simulink model "grid_traditional"  (R2023b)
settings: Solver=ode23s  StartTime=0.0  StopTime=32  RelTol=1e-3
values from neighbouring files (symbols this model uses):
  Ts = 5e-6    (= 5e-06)    [model_parameters.m]
undefined symbols (not defined in the file or in its folder): gcbh, Grid, IBR, L, SG, sps_rtmsupport, TX
libraries: spsThreePhaseVIMeasurementLib x13, spsFourierLib x13, spsPowerPositiveSequenceLib x13, spsThreePhaseSeriesRLCLoadLib x11, spsThreePhaseSeriesRLCBranchLib x10, spsThreePhaseTransformerTwoWindingsLib x10, spsDCVoltageSourceLib x8, spsFirstOrderFilterLib x8, spsabctodq0Lib x8, spsSimplifiedSynchronousMachinepuUnitsLib x6, spsGroundLib x4, spsUniversalBridgeLib x4
(part 2 of 2)

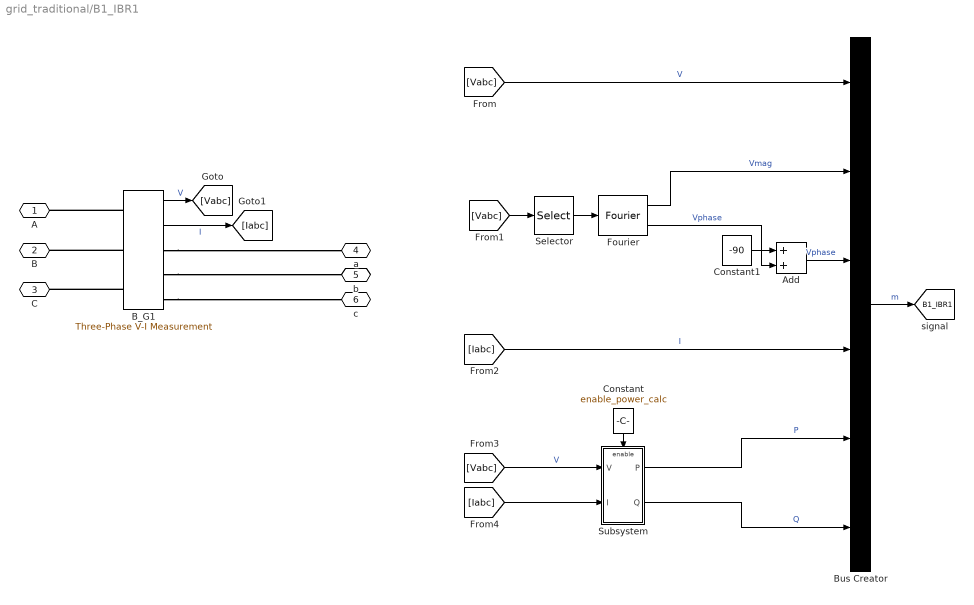
== system grid_traditional/B1_IBR1 ==
  Add : Sum
  B_G1 : spsThreePhaseVIMeasurementLib/Three-Phase V-I Measurement  VoltageMeasurement=phase-to-ground  SetLabelV=off  LabelV=G1_Vabc  Vpu=on  VpuLL=off  CurrentMeasurement=yes  SetLabelI=off  LabelI=G1_Iabc  Ipu=on  Pbase=Sbase  Vbase=Vbase  OutputType=Complex  PhasorSimulation=off  PSBequivalent=0
  Bus Creator : BusCreator  Inputs=6
  Constant : Constant  Value=enable_power_calc  OutDataTypeStr=boolean
  Constant1 : Constant  Value=-90
  Fourier : spsFourierLib/Fourier  Freq=f  n=1  InInit=[0, 0]  Ts=Ts
  Selector : Selector  InputPortWidth=3  IndexOptions=Index vector (dialog)  Indices=[1]  OutputSizes=1
  Subsystem : Subsystem
  A : PMIOPort  Side=Left
  B : PMIOPort  Port=2  Side=Left
  C : PMIOPort  Port=3  Side=Left
  a : PMIOPort  Port=4  Side=Right
  b : PMIOPort  Port=5  Side=Right
  c : PMIOPort  Port=6  Side=Right
  tag scope: B1_IBR1=global
  wires:
  Selector/1 -> Fourier/1
  Bus Creator/1 -> [B1_IBR1]  "m"
  Constant/1 -> Subsystem/Enable
  Subsystem/1(P) -> Bus Creator/5  "P"
  Subsystem/2(Q) -> Bus Creator/6  "Q"
  Fourier/1 -> Bus Creator/2  "Vmag"
  B_G1/1 -> [Vabc]  "V"
  [Vabc] -> Bus Creator/1  "V"
  [Vabc] -> Selector/1
  B_G1/2 -> [Iabc]  "I"
  [Iabc] -> Bus Creator/4  "I"
  [Vabc] -> Subsystem/1(V)  "V"
  [Iabc] -> Subsystem/2(I)
  Add/1 -> Bus Creator/3  "Vphase"
  Fourier/2 -> Add/2  "Vphase"
  Constant1/1 -> Add/1
  connections:
  B_G1/LConn1 -- A/RConn1
  B_G1/LConn3 -- C/RConn1
  B_G1/RConn2 -- b/RConn1
  B_G1/RConn1 -- a/RConn1
  B_G1/LConn2 -- B/RConn1
  B_G1/RConn3 -- c/RConn1

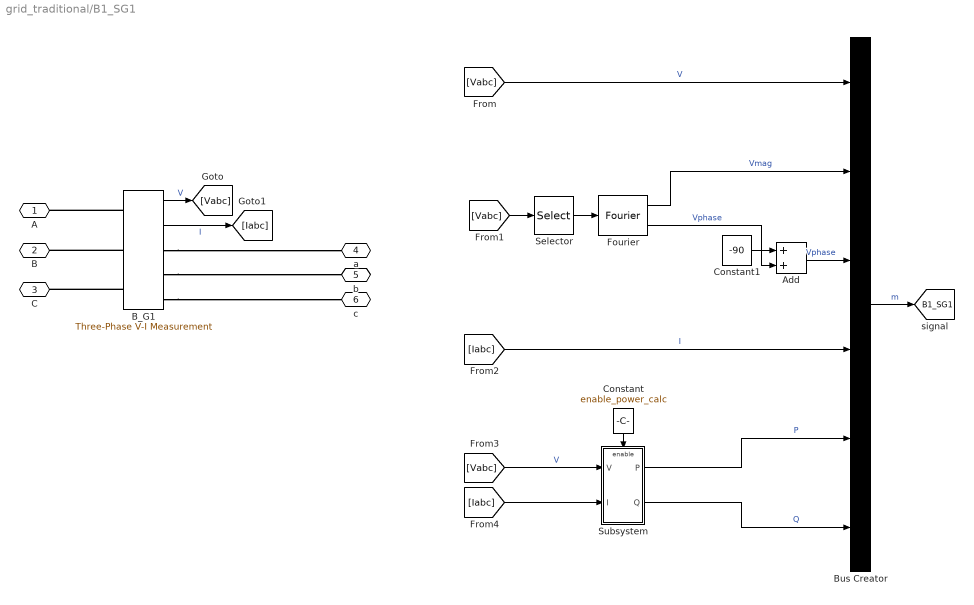
== system grid_traditional/B1_SG1 ==
  Add : Sum
  B_G1 : spsThreePhaseVIMeasurementLib/Three-Phase V-I Measurement  VoltageMeasurement=phase-to-ground  SetLabelV=off  LabelV=G1_Vabc  Vpu=on  VpuLL=off  CurrentMeasurement=yes  SetLabelI=off  LabelI=G1_Iabc  Ipu=on  Pbase=Sbase  Vbase=Vbase  OutputType=Complex  PhasorSimulation=off  PSBequivalent=0
  Bus Creator : BusCreator  Inputs=6
  Constant : Constant  Value=enable_power_calc  OutDataTypeStr=boolean
  Constant1 : Constant  Value=-90
  Fourier : spsFourierLib/Fourier  Freq=f  n=1  InInit=[0, 0]  Ts=Ts
  Selector : Selector  InputPortWidth=3  IndexOptions=Index vector (dialog)  Indices=[1]  OutputSizes=1
  Subsystem : Subsystem
  A : PMIOPort  Side=Left
  B : PMIOPort  Port=2  Side=Left
  C : PMIOPort  Port=3  Side=Left
  a : PMIOPort  Port=4  Side=Right
  b : PMIOPort  Port=5  Side=Right
  c : PMIOPort  Port=6  Side=Right
  tag scope: B1_SG1=global
  wires:
  Selector/1 -> Fourier/1
  Bus Creator/1 -> [B1_SG1]  "m"
  Constant/1 -> Subsystem/Enable
  Subsystem/1(P) -> Bus Creator/5  "P"
  Subsystem/2(Q) -> Bus Creator/6  "Q"
  Fourier/1 -> Bus Creator/2  "Vmag"
  B_G1/1 -> [Vabc]  "V"
  [Vabc] -> Bus Creator/1  "V"
  [Vabc] -> Selector/1
  B_G1/2 -> [Iabc]  "I"
  [Iabc] -> Bus Creator/4  "I"
  [Vabc] -> Subsystem/1(V)  "V"
  [Iabc] -> Subsystem/2(I)
  Add/1 -> Bus Creator/3  "Vphase"
  Fourier/2 -> Add/2  "Vphase"
  Constant1/1 -> Add/1
  connections:
  B_G1/LConn1 -- A/RConn1
  B_G1/LConn3 -- C/RConn1
  B_G1/RConn2 -- b/RConn1
  B_G1/RConn1 -- a/RConn1
  B_G1/LConn2 -- B/RConn1
  B_G1/RConn3 -- c/RConn1

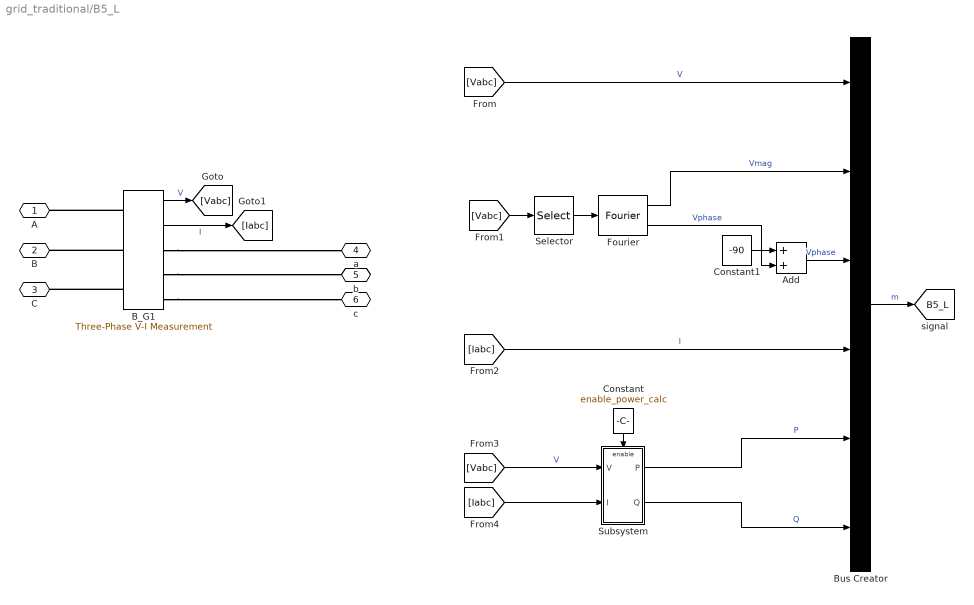
== system grid_traditional/B5_L ==
  Add : Sum
  B_G1 : spsThreePhaseVIMeasurementLib/Three-Phase V-I Measurement  VoltageMeasurement=phase-to-ground  SetLabelV=off  LabelV=G1_Vabc  Vpu=on  VpuLL=off  CurrentMeasurement=yes  SetLabelI=off  LabelI=G1_Iabc  Ipu=on  Pbase=Sbase  Vbase=Vbase  OutputType=Complex  PhasorSimulation=off  PSBequivalent=0
  Bus Creator : BusCreator  Inputs=6
  Constant : Constant  Value=enable_power_calc  OutDataTypeStr=boolean
  Constant1 : Constant  Value=-90
  Fourier : spsFourierLib/Fourier  Freq=f  n=1  InInit=[0, 0]  Ts=Ts
  Selector : Selector  InputPortWidth=3  IndexOptions=Index vector (dialog)  Indices=[1]  OutputSizes=1
  Subsystem : Subsystem
  A : PMIOPort  Side=Left
  B : PMIOPort  Port=2  Side=Left
  C : PMIOPort  Port=3  Side=Left
  a : PMIOPort  Port=4  Side=Right
  b : PMIOPort  Port=5  Side=Right
  c : PMIOPort  Port=6  Side=Right
  tag scope: B5_L=global
  wires:
  Selector/1 -> Fourier/1
  Bus Creator/1 -> [B5_L]  "m"
  Constant/1 -> Subsystem/Enable
  Subsystem/1(P) -> Bus Creator/5  "P"
  Subsystem/2(Q) -> Bus Creator/6  "Q"
  Fourier/1 -> Bus Creator/2  "Vmag"
  B_G1/1 -> [Vabc]  "V"
  [Vabc] -> Bus Creator/1  "V"
  [Vabc] -> Selector/1
  B_G1/2 -> [Iabc]  "I"
  [Iabc] -> Bus Creator/4  "I"
  [Vabc] -> Subsystem/1(V)  "V"
  [Iabc] -> Subsystem/2(I)
  Add/1 -> Bus Creator/3  "Vphase"
  Fourier/2 -> Add/2  "Vphase"
  Constant1/1 -> Add/1
  connections:
  B_G1/LConn1 -- A/RConn1
  B_G1/LConn3 -- C/RConn1
  B_G1/RConn2 -- b/RConn1
  B_G1/RConn1 -- a/RConn1
  B_G1/LConn2 -- B/RConn1
  B_G1/RConn3 -- c/RConn1

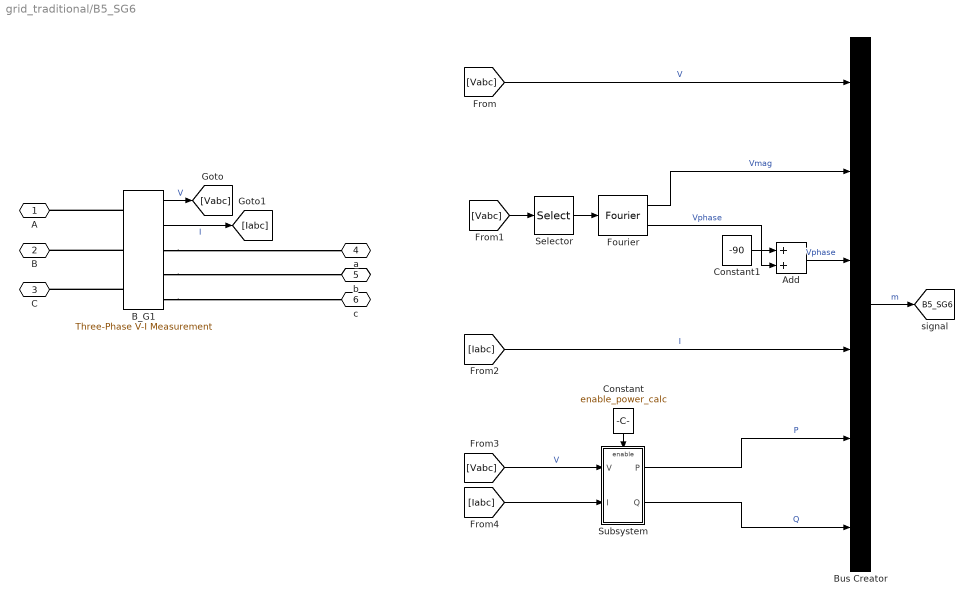
== system grid_traditional/B5_SG6 ==
  Add : Sum
  B_G1 : spsThreePhaseVIMeasurementLib/Three-Phase V-I Measurement  VoltageMeasurement=phase-to-ground  SetLabelV=off  LabelV=G1_Vabc  Vpu=on  VpuLL=off  CurrentMeasurement=yes  SetLabelI=off  LabelI=G1_Iabc  Ipu=on  Pbase=Sbase  Vbase=Vbase  OutputType=Complex  PhasorSimulation=off  PSBequivalent=0
  Bus Creator : BusCreator  Inputs=6
  Constant : Constant  Value=enable_power_calc  OutDataTypeStr=boolean
  Constant1 : Constant  Value=-90
  Fourier : spsFourierLib/Fourier  Freq=f  n=1  InInit=[0, 0]  Ts=Ts
  Selector : Selector  InputPortWidth=3  IndexOptions=Index vector (dialog)  Indices=[1]  OutputSizes=1
  Subsystem : Subsystem
  A : PMIOPort  Side=Left
  B : PMIOPort  Port=2  Side=Left
  C : PMIOPort  Port=3  Side=Left
  a : PMIOPort  Port=4  Side=Right
  b : PMIOPort  Port=5  Side=Right
  c : PMIOPort  Port=6  Side=Right
  tag scope: B5_SG6=global
  wires:
  Selector/1 -> Fourier/1
  Bus Creator/1 -> [B5_SG6]  "m"
  Constant/1 -> Subsystem/Enable
  Subsystem/1(P) -> Bus Creator/5  "P"
  Subsystem/2(Q) -> Bus Creator/6  "Q"
  Fourier/1 -> Bus Creator/2  "Vmag"
  B_G1/1 -> [Vabc]  "V"
  [Vabc] -> Bus Creator/1  "V"
  [Vabc] -> Selector/1
  B_G1/2 -> [Iabc]  "I"
  [Iabc] -> Bus Creator/4  "I"
  [Vabc] -> Subsystem/1(V)  "V"
  [Iabc] -> Subsystem/2(I)
  Add/1 -> Bus Creator/3  "Vphase"
  Fourier/2 -> Add/2  "Vphase"
  Constant1/1 -> Add/1
  connections:
  B_G1/LConn1 -- A/RConn1
  B_G1/LConn3 -- C/RConn1
  B_G1/RConn2 -- b/RConn1
  B_G1/RConn1 -- a/RConn1
  B_G1/LConn2 -- B/RConn1
  B_G1/RConn3 -- c/RConn1

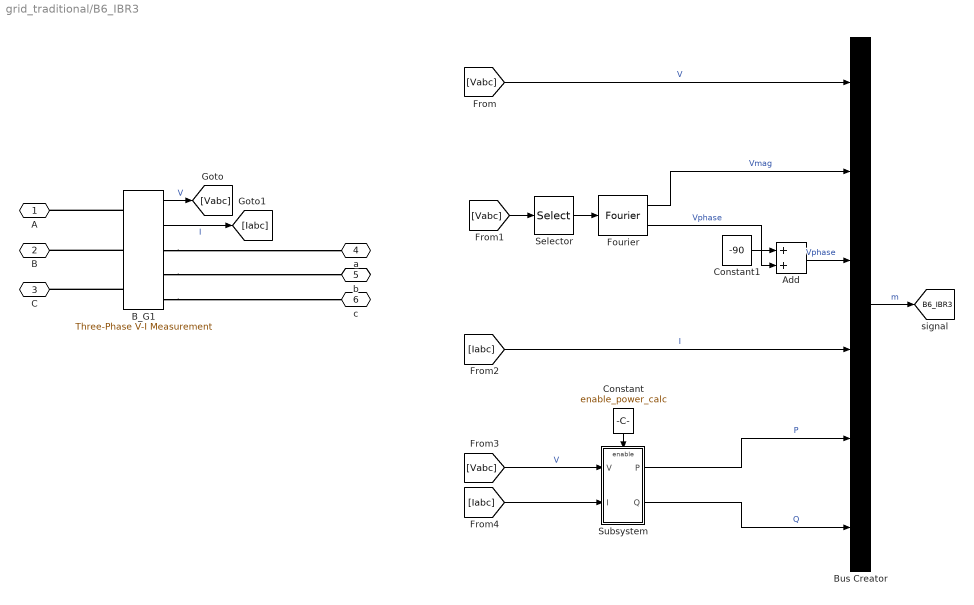
== system grid_traditional/B6_IBR3 ==
  Add : Sum
  B_G1 : spsThreePhaseVIMeasurementLib/Three-Phase V-I Measurement  VoltageMeasurement=phase-to-ground  SetLabelV=off  LabelV=G1_Vabc  Vpu=on  VpuLL=off  CurrentMeasurement=yes  SetLabelI=off  LabelI=G1_Iabc  Ipu=on  Pbase=Sbase  Vbase=Vbase  OutputType=Complex  PhasorSimulation=off  PSBequivalent=0
  Bus Creator : BusCreator  Inputs=6
  Constant : Constant  Value=enable_power_calc  OutDataTypeStr=boolean
  Constant1 : Constant  Value=-90
  Fourier : spsFourierLib/Fourier  Freq=f  n=1  InInit=[0, 0]  Ts=Ts
  Selector : Selector  InputPortWidth=3  IndexOptions=Index vector (dialog)  Indices=[1]  OutputSizes=1
  Subsystem : Subsystem
  A : PMIOPort  Side=Left
  B : PMIOPort  Port=2  Side=Left
  C : PMIOPort  Port=3  Side=Left
  a : PMIOPort  Port=4  Side=Right
  b : PMIOPort  Port=5  Side=Right
  c : PMIOPort  Port=6  Side=Right
  tag scope: B6_IBR3=global
  wires:
  Selector/1 -> Fourier/1
  Bus Creator/1 -> [B6_IBR3]  "m"
  Constant/1 -> Subsystem/Enable
  Subsystem/1(P) -> Bus Creator/5  "P"
  Subsystem/2(Q) -> Bus Creator/6  "Q"
  Fourier/1 -> Bus Creator/2  "Vmag"
  B_G1/1 -> [Vabc]  "V"
  [Vabc] -> Bus Creator/1  "V"
  [Vabc] -> Selector/1
  B_G1/2 -> [Iabc]  "I"
  [Iabc] -> Bus Creator/4  "I"
  [Vabc] -> Subsystem/1(V)  "V"
  [Iabc] -> Subsystem/2(I)
  Add/1 -> Bus Creator/3  "Vphase"
  Fourier/2 -> Add/2  "Vphase"
  Constant1/1 -> Add/1
  connections:
  B_G1/LConn1 -- A/RConn1
  B_G1/LConn3 -- C/RConn1
  B_G1/RConn2 -- b/RConn1
  B_G1/RConn1 -- a/RConn1
  B_G1/LConn2 -- B/RConn1
  B_G1/RConn3 -- c/RConn1

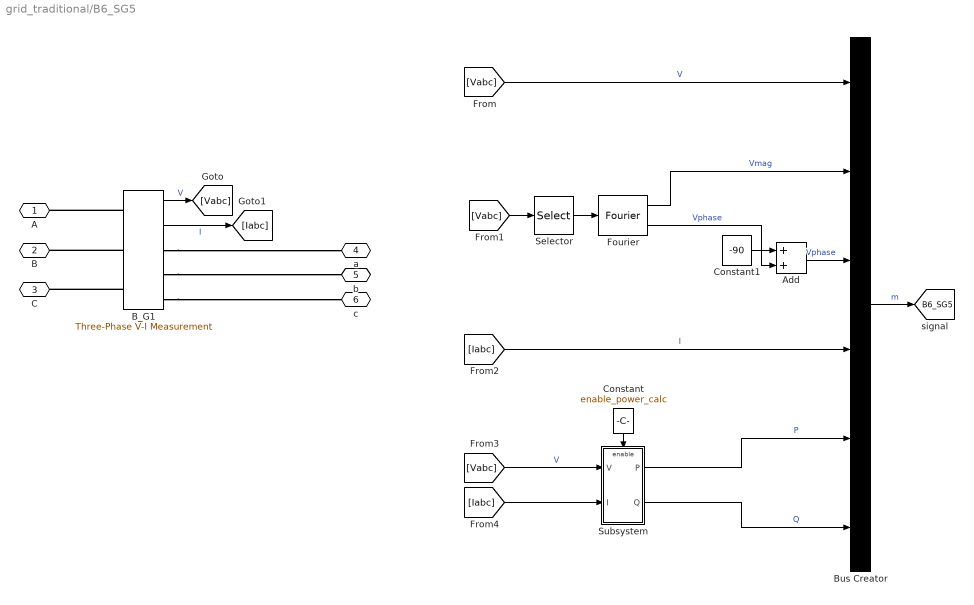
== system grid_traditional/B6_SG5 ==
  Add : Sum
  B_G1 : spsThreePhaseVIMeasurementLib/Three-Phase V-I Measurement  VoltageMeasurement=phase-to-ground  SetLabelV=off  LabelV=G1_Vabc  Vpu=on  VpuLL=off  CurrentMeasurement=yes  SetLabelI=off  LabelI=G1_Iabc  Ipu=on  Pbase=Sbase  Vbase=Vbase  OutputType=Complex  PhasorSimulation=off  PSBequivalent=0
  Bus Creator : BusCreator  Inputs=6
  Constant : Constant  Value=enable_power_calc  OutDataTypeStr=boolean
  Constant1 : Constant  Value=-90
  Fourier : spsFourierLib/Fourier  Freq=f  n=1  InInit=[0, 0]  Ts=Ts
  Selector : Selector  InputPortWidth=3  IndexOptions=Index vector (dialog)  Indices=[1]  OutputSizes=1
  Subsystem : Subsystem
  A : PMIOPort  Side=Left
  B : PMIOPort  Port=2  Side=Left
  C : PMIOPort  Port=3  Side=Left
  a : PMIOPort  Port=4  Side=Right
  b : PMIOPort  Port=5  Side=Right
  c : PMIOPort  Port=6  Side=Right
  tag scope: B6_SG5=global
  wires:
  Selector/1 -> Fourier/1
  Bus Creator/1 -> [B6_SG5]  "m"
  Constant/1 -> Subsystem/Enable
  Subsystem/1(P) -> Bus Creator/5  "P"
  Subsystem/2(Q) -> Bus Creator/6  "Q"
  Fourier/1 -> Bus Creator/2  "Vmag"
  B_G1/1 -> [Vabc]  "V"
  [Vabc] -> Bus Creator/1  "V"
  [Vabc] -> Selector/1
  B_G1/2 -> [Iabc]  "I"
  [Iabc] -> Bus Creator/4  "I"
  [Vabc] -> Subsystem/1(V)  "V"
  [Iabc] -> Subsystem/2(I)
  Add/1 -> Bus Creator/3  "Vphase"
  Fourier/2 -> Add/2  "Vphase"
  Constant1/1 -> Add/1
  connections:
  B_G1/LConn1 -- A/RConn1
  B_G1/LConn3 -- C/RConn1
  B_G1/RConn2 -- b/RConn1
  B_G1/RConn1 -- a/RConn1
  B_G1/LConn2 -- B/RConn1
  B_G1/RConn3 -- c/RConn1

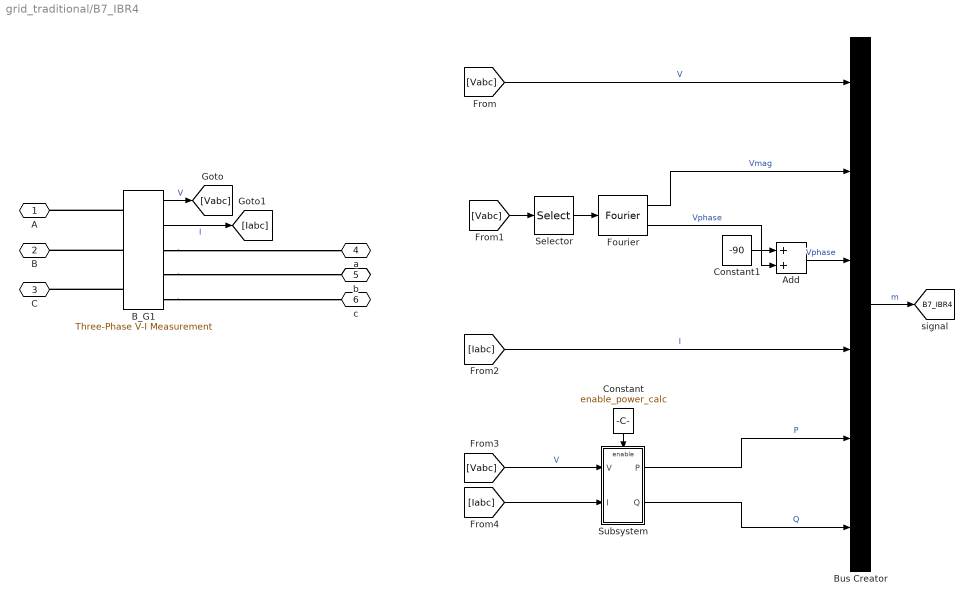
== system grid_traditional/B7_IBR4 ==
  Add : Sum
  B_G1 : spsThreePhaseVIMeasurementLib/Three-Phase V-I Measurement  VoltageMeasurement=phase-to-ground  SetLabelV=off  LabelV=G1_Vabc  Vpu=on  VpuLL=off  CurrentMeasurement=yes  SetLabelI=off  LabelI=G1_Iabc  Ipu=on  Pbase=Sbase  Vbase=Vbase  OutputType=Complex  PhasorSimulation=off  PSBequivalent=0
  Bus Creator : BusCreator  Inputs=6
  Constant : Constant  Value=enable_power_calc  OutDataTypeStr=boolean
  Constant1 : Constant  Value=-90
  Fourier : spsFourierLib/Fourier  Freq=f  n=1  InInit=[0, 0]  Ts=Ts
  Selector : Selector  InputPortWidth=3  IndexOptions=Index vector (dialog)  Indices=[1]  OutputSizes=1
  Subsystem : Subsystem
  A : PMIOPort  Side=Left
  B : PMIOPort  Port=2  Side=Left
  C : PMIOPort  Port=3  Side=Left
  a : PMIOPort  Port=4  Side=Right
  b : PMIOPort  Port=5  Side=Right
  c : PMIOPort  Port=6  Side=Right
  tag scope: B7_IBR4=global
  wires:
  Selector/1 -> Fourier/1
  Bus Creator/1 -> [B7_IBR4]  "m"
  Constant/1 -> Subsystem/Enable
  Subsystem/1(P) -> Bus Creator/5  "P"
  Subsystem/2(Q) -> Bus Creator/6  "Q"
  Fourier/1 -> Bus Creator/2  "Vmag"
  B_G1/1 -> [Vabc]  "V"
  [Vabc] -> Bus Creator/1  "V"
  [Vabc] -> Selector/1
  B_G1/2 -> [Iabc]  "I"
  [Iabc] -> Bus Creator/4  "I"
  [Vabc] -> Subsystem/1(V)  "V"
  [Iabc] -> Subsystem/2(I)
  Add/1 -> Bus Creator/3  "Vphase"
  Fourier/2 -> Add/2  "Vphase"
  Constant1/1 -> Add/1
  connections:
  B_G1/LConn1 -- A/RConn1
  B_G1/LConn3 -- C/RConn1
  B_G1/RConn2 -- b/RConn1
  B_G1/RConn1 -- a/RConn1
  B_G1/LConn2 -- B/RConn1
  B_G1/RConn3 -- c/RConn1

== system grid_traditional/B7_L ==
  Add : Sum
  B_G1 : spsThreePhaseVIMeasurementLib/Three-Phase V-I Measurement  VoltageMeasurement=phase-to-ground  SetLabelV=off  LabelV=G1_Vabc  Vpu=on  VpuLL=off  CurrentMeasurement=yes  SetLabelI=off  LabelI=G1_Iabc  Ipu=on  Pbase=Sbase  Vbase=Vbase  OutputType=Complex  PhasorSimulation=off  PSBequivalent=0
  Bus Creator : BusCreator  Inputs=6
  Constant : Constant  Value=enable_power_calc  OutDataTypeStr=boolean
  Constant1 : Constant  Value=-90
  Fourier : spsFourierLib/Fourier  Freq=f  n=1  InInit=[0, 0]  Ts=Ts
  Selector : Selector  InputPortWidth=3  IndexOptions=Index vector (dialog)  Indices=[1]  OutputSizes=1
  Subsystem : Subsystem
  A : PMIOPort  Side=Left
  B : PMIOPort  Port=2  Side=Left
  C : PMIOPort  Port=3  Side=Left
  a : PMIOPort  Port=4  Side=Right
  b : PMIOPort  Port=5  Side=Right
  c : PMIOPort  Port=6  Side=Right
  tag scope: B7_L=global
  wires:
  Selector/1 -> Fourier/1
  Bus Creator/1 -> [B7_L]  "m"
  Constant/1 -> Subsystem/Enable
  Subsystem/1(P) -> Bus Creator/5  "P"
  Subsystem/2(Q) -> Bus Creator/6  "Q"
  Fourier/1 -> Bus Creator/2  "Vmag"
  B_G1/1 -> [Vabc]  "V"
  [Vabc] -> Bus Creator/1  "V"
  [Vabc] -> Selector/1
  B_G1/2 -> [Iabc]  "I"
  [Iabc] -> Bus Creator/4  "I"
  [Vabc] -> Subsystem/1(V)  "V"
  [Iabc] -> Subsystem/2(I)
  Add/1 -> Bus Creator/3  "Vphase"
  Fourier/2 -> Add/2  "Vphase"
  Constant1/1 -> Add/1
  connections:
  B_G1/LConn1 -- A/RConn1
  B_G1/LConn3 -- C/RConn1
  B_G1/RConn2 -- b/RConn1
  B_G1/RConn1 -- a/RConn1
  B_G1/LConn2 -- B/RConn1
  B_G1/RConn3 -- c/RConn1

== system grid_traditional/B7_SG4 ==
  Add : Sum
  B_G1 : spsThreePhaseVIMeasurementLib/Three-Phase V-I Measurement  VoltageMeasurement=phase-to-ground  SetLabelV=off  LabelV=G1_Vabc  Vpu=on  VpuLL=off  CurrentMeasurement=yes  SetLabelI=off  LabelI=G1_Iabc  Ipu=on  Pbase=Sbase  Vbase=Vbase  OutputType=Complex  PhasorSimulation=off  PSBequivalent=0
  Bus Creator : BusCreator  Inputs=6
  Constant : Constant  Value=enable_power_calc  OutDataTypeStr=boolean
  Constant1 : Constant  Value=-90
  Fourier : spsFourierLib/Fourier  Freq=f  n=1  InInit=[0, 0]  Ts=Ts
  Selector : Selector  InputPortWidth=3  IndexOptions=Index vector (dialog)  Indices=[1]  OutputSizes=1
  Subsystem : Subsystem
  A : PMIOPort  Side=Left
  B : PMIOPort  Port=2  Side=Left
  C : PMIOPort  Port=3  Side=Left
  a : PMIOPort  Port=4  Side=Right
  b : PMIOPort  Port=5  Side=Right
  c : PMIOPort  Port=6  Side=Right
  tag scope: B7_SG4=global
  wires:
  Selector/1 -> Fourier/1
  Bus Creator/1 -> [B7_SG4]  "m"
  Constant/1 -> Subsystem/Enable
  Subsystem/1(P) -> Bus Creator/5  "P"
  Subsystem/2(Q) -> Bus Creator/6  "Q"
  Fourier/1 -> Bus Creator/2  "Vmag"
  B_G1/1 -> [Vabc]  "V"
  [Vabc] -> Bus Creator/1  "V"
  [Vabc] -> Selector/1
  B_G1/2 -> [Iabc]  "I"
  [Iabc] -> Bus Creator/4  "I"
  [Vabc] -> Subsystem/1(V)  "V"
  [Iabc] -> Subsystem/2(I)
  Add/1 -> Bus Creator/3  "Vphase"
  Fourier/2 -> Add/2  "Vphase"
  Constant1/1 -> Add/1
  connections:
  B_G1/LConn1 -- A/RConn1
  B_G1/LConn3 -- C/RConn1
  B_G1/RConn2 -- b/RConn1
  B_G1/RConn1 -- a/RConn1
  B_G1/LConn2 -- B/RConn1
  B_G1/RConn3 -- c/RConn1

== system grid_traditional/B8_IBR2 ==
  Add : Sum
  B_G1 : spsThreePhaseVIMeasurementLib/Three-Phase V-I Measurement  VoltageMeasurement=phase-to-ground  SetLabelV=off  LabelV=G1_Vabc  Vpu=on  VpuLL=off  CurrentMeasurement=yes  SetLabelI=off  LabelI=G1_Iabc  Ipu=on  Pbase=Sbase  Vbase=Vbase  OutputType=Complex  PhasorSimulation=off  PSBequivalent=0
  Bus Creator : BusCreator  Inputs=6
  Constant : Constant  Value=enable_power_calc  OutDataTypeStr=boolean
  Constant1 : Constant  Value=-90
  Fourier : spsFourierLib/Fourier  Freq=f  n=1  InInit=[0, 0]  Ts=Ts
  Selector : Selector  InputPortWidth=3  IndexOptions=Index vector (dialog)  Indices=[1]  OutputSizes=1
  Subsystem : Subsystem
  A : PMIOPort  Side=Left
  B : PMIOPort  Port=2  Side=Left
  C : PMIOPort  Port=3  Side=Left
  a : PMIOPort  Port=4  Side=Right
  b : PMIOPort  Port=5  Side=Right
  c : PMIOPort  Port=6  Side=Right
  tag scope: B8_IBR2=global
  wires:
  Selector/1 -> Fourier/1
  Bus Creator/1 -> [B8_IBR2]  "m"
  Constant/1 -> Subsystem/Enable
  Subsystem/1(P) -> Bus Creator/5  "P"
  Subsystem/2(Q) -> Bus Creator/6  "Q"
  Fourier/1 -> Bus Creator/2  "Vmag"
  B_G1/1 -> [Vabc]  "V"
  [Vabc] -> Bus Creator/1  "V"
  [Vabc] -> Selector/1
  B_G1/2 -> [Iabc]  "I"
  [Iabc] -> Bus Creator/4  "I"
  [Vabc] -> Subsystem/1(V)  "V"
  [Iabc] -> Subsystem/2(I)
  Add/1 -> Bus Creator/3  "Vphase"
  Fourier/2 -> Add/2  "Vphase"
  Constant1/1 -> Add/1
  connections:
  B_G1/LConn1 -- A/RConn1
  B_G1/LConn3 -- C/RConn1
  B_G1/RConn2 -- b/RConn1
  B_G1/RConn1 -- a/RConn1
  B_G1/LConn2 -- B/RConn1
  B_G1/RConn3 -- c/RConn1

== system grid_traditional/B8_SG3 ==
  Add : Sum
  B_G1 : spsThreePhaseVIMeasurementLib/Three-Phase V-I Measurement  VoltageMeasurement=phase-to-ground  SetLabelV=off  LabelV=G1_Vabc  Vpu=on  VpuLL=off  CurrentMeasurement=yes  SetLabelI=off  LabelI=G1_Iabc  Ipu=on  Pbase=Sbase  Vbase=Vbase  OutputType=Complex  PhasorSimulation=off  PSBequivalent=0
  Bus Creator : BusCreator  Inputs=6
  Constant : Constant  Value=enable_power_calc  OutDataTypeStr=boolean
  Constant1 : Constant  Value=-90
  Fourier : spsFourierLib/Fourier  Freq=f  n=1  InInit=[0, 0]  Ts=Ts
  Selector : Selector  InputPortWidth=3  IndexOptions=Index vector (dialog)  Indices=[1]  OutputSizes=1
  Subsystem : Subsystem
  A : PMIOPort  Side=Left
  B : PMIOPort  Port=2  Side=Left
  C : PMIOPort  Port=3  Side=Left
  a : PMIOPort  Port=4  Side=Right
  b : PMIOPort  Port=5  Side=Right
  c : PMIOPort  Port=6  Side=Right
  tag scope: B8_SG3=global
  wires:
  Selector/1 -> Fourier/1
  Bus Creator/1 -> [B8_SG3]  "m"
  Constant/1 -> Subsystem/Enable
  Subsystem/1(P) -> Bus Creator/5  "P"
  Subsystem/2(Q) -> Bus Creator/6  "Q"
  Fourier/1 -> Bus Creator/2  "Vmag"
  B_G1/1 -> [Vabc]  "V"
  [Vabc] -> Bus Creator/1  "V"
  [Vabc] -> Selector/1
  B_G1/2 -> [Iabc]  "I"
  [Iabc] -> Bus Creator/4  "I"
  [Vabc] -> Subsystem/1(V)  "V"
  [Iabc] -> Subsystem/2(I)
  Add/1 -> Bus Creator/3  "Vphase"
  Fourier/2 -> Add/2  "Vphase"
  Constant1/1 -> Add/1
  connections:
  B_G1/LConn1 -- A/RConn1
  B_G1/LConn3 -- C/RConn1
  B_G1/RConn2 -- b/RConn1
  B_G1/RConn1 -- a/RConn1
  B_G1/LConn2 -- B/RConn1
  B_G1/RConn3 -- c/RConn1

== system grid_traditional/B9_L ==
  Add : Sum
  B_G1 : spsThreePhaseVIMeasurementLib/Three-Phase V-I Measurement  VoltageMeasurement=phase-to-ground  SetLabelV=off  LabelV=G1_Vabc  Vpu=on  VpuLL=off  CurrentMeasurement=yes  SetLabelI=off  LabelI=G1_Iabc  Ipu=on  Pbase=Sbase  Vbase=Vbase  OutputType=Complex  PhasorSimulation=off  PSBequivalent=0
  Bus Creator : BusCreator  Inputs=6
  Constant : Constant  Value=enable_power_calc  OutDataTypeStr=boolean
  Constant1 : Constant  Value=-90
  Fourier : spsFourierLib/Fourier  Freq=f  n=1  InInit=[0, 0]  Ts=Ts
  Selector : Selector  InputPortWidth=3  IndexOptions=Index vector (dialog)  Indices=[1]  OutputSizes=1
  Subsystem : Subsystem
  A : PMIOPort  Side=Left
  B : PMIOPort  Port=2  Side=Left
  C : PMIOPort  Port=3  Side=Left
  a : PMIOPort  Port=4  Side=Right
  b : PMIOPort  Port=5  Side=Right
  c : PMIOPort  Port=6  Side=Right
  tag scope: B9_L=global
  wires:
  Selector/1 -> Fourier/1
  Bus Creator/1 -> [B9_L]  "m"
  Constant/1 -> Subsystem/Enable
  Subsystem/1(P) -> Bus Creator/5  "P"
  Subsystem/2(Q) -> Bus Creator/6  "Q"
  Fourier/1 -> Bus Creator/2  "Vmag"
  B_G1/1 -> [Vabc]  "V"
  [Vabc] -> Bus Creator/1  "V"
  [Vabc] -> Selector/1
  B_G1/2 -> [Iabc]  "I"
  [Iabc] -> Bus Creator/4  "I"
  [Vabc] -> Subsystem/1(V)  "V"
  [Iabc] -> Subsystem/2(I)
  Add/1 -> Bus Creator/3  "Vphase"
  Fourier/2 -> Add/2  "Vphase"
  Constant1/1 -> Add/1
  connections:
  B_G1/LConn1 -- A/RConn1
  B_G1/LConn3 -- C/RConn1
  B_G1/RConn2 -- b/RConn1
  B_G1/RConn1 -- a/RConn1
  B_G1/LConn2 -- B/RConn1
  B_G1/RConn3 -- c/RConn1

== system grid_traditional/B9_SG2 ==
  Add : Sum
  B_G1 : spsThreePhaseVIMeasurementLib/Three-Phase V-I Measurement  VoltageMeasurement=phase-to-ground  SetLabelV=off  LabelV=G1_Vabc  Vpu=on  VpuLL=off  CurrentMeasurement=yes  SetLabelI=off  LabelI=G1_Iabc  Ipu=on  Pbase=Sbase  Vbase=Vbase  OutputType=Complex  PhasorSimulation=off  PSBequivalent=0
  Bus Creator : BusCreator  Inputs=6
  Constant : Constant  Value=enable_power_calc  OutDataTypeStr=boolean
  Constant1 : Constant  Value=-90
  Fourier : spsFourierLib/Fourier  Freq=f  n=1  InInit=[0, 0]  Ts=Ts
  Selector : Selector  InputPortWidth=3  IndexOptions=Index vector (dialog)  Indices=[1]  OutputSizes=1
  Subsystem : Subsystem
  A : PMIOPort  Side=Left
  B : PMIOPort  Port=2  Side=Left
  C : PMIOPort  Port=3  Side=Left
  a : PMIOPort  Port=4  Side=Right
  b : PMIOPort  Port=5  Side=Right
  c : PMIOPort  Port=6  Side=Right
  tag scope: B9_SG2=global
  wires:
  Selector/1 -> Fourier/1
  Bus Creator/1 -> [B9_SG2]  "m"
  Constant/1 -> Subsystem/Enable
  Subsystem/1(P) -> Bus Creator/5  "P"
  Subsystem/2(Q) -> Bus Creator/6  "Q"
  Fourier/1 -> Bus Creator/2  "Vmag"
  B_G1/1 -> [Vabc]  "V"
  [Vabc] -> Bus Creator/1  "V"
  [Vabc] -> Selector/1
  B_G1/2 -> [Iabc]  "I"
  [Iabc] -> Bus Creator/4  "I"
  [Vabc] -> Subsystem/1(V)  "V"
  [Iabc] -> Subsystem/2(I)
  Add/1 -> Bus Creator/3  "Vphase"
  Fourier/2 -> Add/2  "Vphase"
  Constant1/1 -> Add/1
  connections:
  B_G1/LConn1 -- A/RConn1
  B_G1/LConn3 -- C/RConn1
  B_G1/RConn2 -- b/RConn1
  B_G1/RConn1 -- a/RConn1
  B_G1/LConn2 -- B/RConn1
  B_G1/RConn3 -- c/RConn1

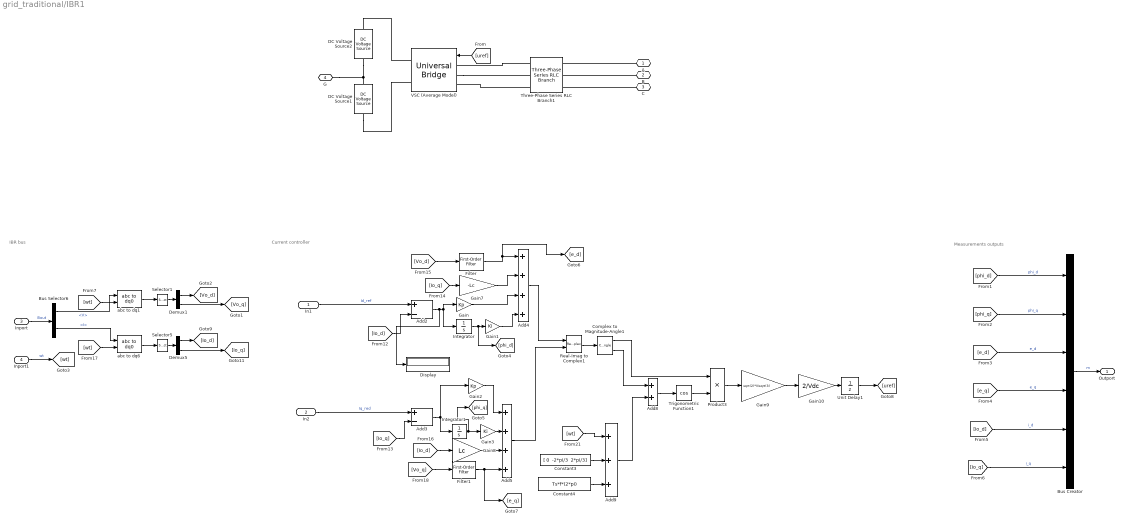
== system grid_traditional/IBR1 ==
  note: IBR bus
  note: Current controller
  note: Measurements outputs
  In1 : Inport
  In2 : Inport  Port=2
  Inport : Inport  Port=3
  Inport1 : Inport  Port=4
  Add2 : Sum  Inputs=+-
  Add3 : Sum  Inputs=+-
  Add4 : Sum  Inputs=++++
  Add5 : Sum  Inputs=++++
  Add8 : Sum
  Add9 : Sum  Inputs=+++
  Bus Creator : BusCreator  Inputs=6
  Bus Selector6 : BusSelector  OutputSignals=V,I
  Complex to Magnitude-Angle1 : ComplexToMagnitudeAngle
  Constant3 : Constant  Value="[ 0  -2*pi/3  2*pi/3]"
  Constant4 : Constant  Value=Ts*f*(2*pi)
  DC Voltage Source1 : spsDCVoltageSourceLib/DC Voltage Source  Amplitude=Vdc/2  Measurements=None
  DC Voltage Source2 : spsDCVoltageSourceLib/DC Voltage Source  Amplitude=Vdc/2  Measurements=None
  Demux1 : Demux  Outputs=2
  Demux5 : Demux  Outputs=2
  Display : Display
  Filter : spsFirstOrderFilterLib/First-Order Filter  FilterType=Lowpass  Tc=Tf  Ts=Ts  Initialize=on  Vac_Init=[0, 0, f]  Vdc_Init=0  PlotResponse=off  FreqRange="[0,  200,  1]"
  Filter1 : spsFirstOrderFilterLib/First-Order Filter  FilterType=Lowpass  Tc=Tf  Ts=Ts  Initialize=on  Vac_Init=[0, 0, f]  Vdc_Init=0  PlotResponse=off  FreqRange="[0,  200,  1]"
  Gain : Gain  Gain=Kp
  Gain1 : Gain  Gain=Ki
  Gain10 : Gain  Gain=2/Vdc
  Gain2 : Gain  Gain=Kp
  Gain3 : Gain  Gain=Ki
  Gain7 : Gain  Gain=-Lc
  Gain8 : Gain  Gain=Lc
  Gain9 : Gain  Gain=sqrt(2)*V/sqrt(3)
  Integrator : Integrator
  Integrator1 : Integrator
  Product3 : Product  Inputs=**  RndMeth=Zero
  Real-Imag to Complex1 : RealImagToComplex
  Selector1 : Selector  InputPortWidth=3  IndexOptions=Index vector (dialog)  Indices=[1 2]  OutputSizes=1
  Selector5 : Selector  InputPortWidth=3  IndexOptions=Index vector (dialog)  Indices=[1 2]  OutputSizes=1
  Three-Phase Series RLC Branch1 : spsThreePhaseSeriesRLCBranchLib/Three-Phase Series RLC Branch  LConnTagsString=A|B|C  RConnTagsString=A|B|C  BranchType=RL  Resistance=Rf*V^2/S  Inductance=Lf*V^2/S*1/(2*pi*f)  Capacitance=1e-6  Measurements=None
  Trigonometric Function1 : Trigonometry  Operator=cos
  Unit Delay1 : UnitDelay  SampleTime=Ts  HasFrameUpgradeWarning=on
  VSC (Average Model) : spsUniversalBridgeLib/Universal Bridge  Arms=3  SnubberResistance=1e5  SnubberCapacitance=inf  Device=Average-model based VSC  Ron=1e-3  Lon=0  ForwardVoltages="[  0  0  ]"  ForwardVoltage=0  GTOparameters=[ 10e-6 , 20e-6 ]  IGBTparameters=[ 1e-6 , 2e-6 ]  Measurements=None  Measurements_2=None  converterType=Rectifier
  abc to dq1 : spsabctodq0Lib/abc to dq0  Alignment=Aligned with phase A axis
  abc to dq6 : spsabctodq0Lib/abc to dq0  Alignment=Aligned with phase A axis
  A : PMIOPort  Side=Right
  B : PMIOPort  Port=2  Side=Right
  C : PMIOPort  Port=3  Side=Right
  G : PMIOPort  Port=4  Side=Left
  Outport : Outport
  wires:
  Add8/1 -> Trigonometric Function1/1
  [uref] -> VSC (Average Model)/1
  Add5/1 -> Real-Imag to Complex1/2
  Constant3/1 -> Add9/2
  Gain9/1 -> Gain10/1
  Gain7/1 -> Add4/2
  Unit Delay1/1 -> [uref]
  Trigonometric Function1/1 -> Product3/2
  [wt] -> Add9/1
  Complex to Magnitude-Angle1/2 -> Add8/1
  Add2/1 -> Display/1, Gain/1, Integrator/1
  Selector5/1 -> Demux5/1
  Demux5/2 -> [Io_q]
  [wt] -> abc to dq6/2
  Filter/1 -> [e_d], Add4/1
  [Vo_q] -> Filter1/1
  Product3/1 -> Gain9/1
  Bus Selector6/2 -> abc to dq6/1  "<I>"
  [Io_d] -> Add2/2
  [Io_q] -> Add3/2
  [Vo_d] -> Filter/1
  Add4/1 -> Real-Imag to Complex1/1
  Real-Imag to Complex1/1 -> Complex to Magnitude-Angle1/1
  [Io_q] -> Gain7/1
  Complex to Magnitude-Angle1/1 -> Product3/1
  abc to dq6/1 -> Selector5/1
  In1/1 -> Add2/1  "Id_ref"
  Add9/1 -> Add8/2
  In2/1 -> Add3/1  "Iq_red"
  Constant4/1 -> Add9/3
  [Io_d] -> Gain8/1
  Gain/1 -> Add4/3
  Inport/1 -> Bus Selector6/1  "Bout"
  Gain10/1 -> Unit Delay1/1
  Demux5/1 -> [Io_d]
  Bus Creator/1 -> Outport/1  "m"
  [phi_d] -> Bus Creator/1  "phi_d"
  [phi_q] -> Bus Creator/2  "phi_q"
  [e_d] -> Bus Creator/3  "e_d"
  [e_q] -> Bus Creator/4  "e_q"
  [Io_d] -> Bus Creator/5  "i_d"
  [Io_q] -> Bus Creator/6  "i_q"
  Inport1/1 -> [wt]  "wt"
  Integrator/1 -> [phi_d], Gain1/1
  Gain1/1 -> Add4/4
  Integrator1/1 -> Gain3/1, [phi_q]
  Filter1/1 -> [e_q], Add5/4
  Gain8/1 -> Add5/3
  Gain2/1 -> Add5/1
  Add3/1 -> Integrator1/1, Gain2/1
  Gain3/1 -> Add5/2
  abc to dq1/1 -> Selector1/1
  Demux1/1 -> [Vo_d]
  Selector1/1 -> Demux1/1
  Demux1/2 -> [Vo_q]
  Bus Selector6/1 -> abc to dq1/1  "<V>"
  [wt] -> abc to dq1/2
  connections:
  A/RConn1 -- Three-Phase Series RLC Branch1/RConn1
  C/RConn1 -- Three-Phase Series RLC Branch1/RConn3
  DC Voltage Source2/LConn1 -- G/RConn1 -- DC Voltage Source1/RConn1
  Three-Phase Series RLC Branch1/LConn1 -- VSC (Average Model)/LConn1
  DC Voltage Source1/LConn1 -- VSC (Average Model)/RConn2
  B/RConn1 -- Three-Phase Series RLC Branch1/RConn2
  VSC (Average Model)/RConn1 -- DC Voltage Source2/RConn1
  Three-Phase Series RLC Branch1/LConn3 -- VSC (Average Model)/LConn3
  VSC (Average Model)/LConn2 -- Three-Phase Series RLC Branch1/LConn2

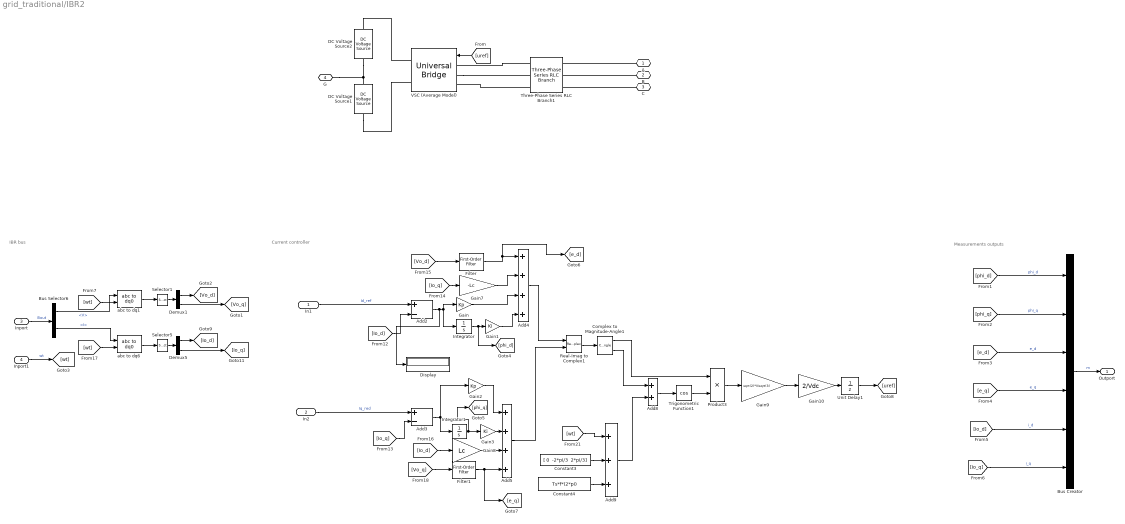
== system grid_traditional/IBR2 ==
  note: IBR bus
  note: Current controller
  note: Measurements outputs
  In1 : Inport
  In2 : Inport  Port=2
  Inport : Inport  Port=3
  Inport1 : Inport  Port=4
  Add2 : Sum  Inputs=+-
  Add3 : Sum  Inputs=+-
  Add4 : Sum  Inputs=++++
  Add5 : Sum  Inputs=++++
  Add8 : Sum
  Add9 : Sum  Inputs=+++
  Bus Creator : BusCreator  Inputs=6
  Bus Selector6 : BusSelector  OutputSignals=V,I
  Complex to Magnitude-Angle1 : ComplexToMagnitudeAngle
  Constant3 : Constant  Value="[ 0  -2*pi/3  2*pi/3]"
  Constant4 : Constant  Value=Ts*f*(2*pi)
  DC Voltage Source1 : spsDCVoltageSourceLib/DC Voltage Source  Amplitude=Vdc/2  Measurements=None
  DC Voltage Source2 : spsDCVoltageSourceLib/DC Voltage Source  Amplitude=Vdc/2  Measurements=None
  Demux1 : Demux  Outputs=2
  Demux5 : Demux  Outputs=2
  Display : Display
  Filter : spsFirstOrderFilterLib/First-Order Filter  FilterType=Lowpass  Tc=Tf  Ts=Ts  Initialize=on  Vac_Init=[0, 0, f]  Vdc_Init=0  PlotResponse=off  FreqRange="[0,  200,  1]"
  Filter1 : spsFirstOrderFilterLib/First-Order Filter  FilterType=Lowpass  Tc=Tf  Ts=Ts  Initialize=on  Vac_Init=[0, 0, f]  Vdc_Init=0  PlotResponse=off  FreqRange="[0,  200,  1]"
  Gain : Gain  Gain=Kp
  Gain1 : Gain  Gain=Ki
  Gain10 : Gain  Gain=2/Vdc
  Gain2 : Gain  Gain=Kp
  Gain3 : Gain  Gain=Ki
  Gain7 : Gain  Gain=-Lc
  Gain8 : Gain  Gain=Lc
  Gain9 : Gain  Gain=sqrt(2)*V/sqrt(3)
  Integrator : Integrator
  Integrator1 : Integrator
  Product3 : Product  Inputs=**  RndMeth=Zero
  Real-Imag to Complex1 : RealImagToComplex
  Selector1 : Selector  InputPortWidth=3  IndexOptions=Index vector (dialog)  Indices=[1 2]  OutputSizes=1
  Selector5 : Selector  InputPortWidth=3  IndexOptions=Index vector (dialog)  Indices=[1 2]  OutputSizes=1
  Three-Phase Series RLC Branch1 : spsThreePhaseSeriesRLCBranchLib/Three-Phase Series RLC Branch  LConnTagsString=A|B|C  RConnTagsString=A|B|C  BranchType=RL  Resistance=Rf*V^2/S  Inductance=Lf*V^2/S*1/(2*pi*f)  Capacitance=1e-6  Measurements=None
  Trigonometric Function1 : Trigonometry  Operator=cos
  Unit Delay1 : UnitDelay  SampleTime=Ts  HasFrameUpgradeWarning=on
  VSC (Average Model) : spsUniversalBridgeLib/Universal Bridge  Arms=3  SnubberResistance=1e5  SnubberCapacitance=inf  Device=Average-model based VSC  Ron=1e-3  Lon=0  ForwardVoltages="[  0  0  ]"  ForwardVoltage=0  GTOparameters=[ 10e-6 , 20e-6 ]  IGBTparameters=[ 1e-6 , 2e-6 ]  Measurements=None  Measurements_2=None  converterType=Rectifier
  abc to dq1 : spsabctodq0Lib/abc to dq0  Alignment=Aligned with phase A axis
  abc to dq6 : spsabctodq0Lib/abc to dq0  Alignment=Aligned with phase A axis
  A : PMIOPort  Side=Right
  B : PMIOPort  Port=2  Side=Right
  C : PMIOPort  Port=3  Side=Right
  G : PMIOPort  Port=4  Side=Left
  Outport : Outport
  wires:
  Add8/1 -> Trigonometric Function1/1
  [uref] -> VSC (Average Model)/1
  Add5/1 -> Real-Imag to Complex1/2
  Constant3/1 -> Add9/2
  Gain9/1 -> Gain10/1
  Gain7/1 -> Add4/2
  Unit Delay1/1 -> [uref]
  Trigonometric Function1/1 -> Product3/2
  [wt] -> Add9/1
  Complex to Magnitude-Angle1/2 -> Add8/1
  Add2/1 -> Display/1, Gain/1, Integrator/1
  Selector5/1 -> Demux5/1
  Demux5/2 -> [Io_q]
  [wt] -> abc to dq6/2
  Filter/1 -> [e_d], Add4/1
  [Vo_q] -> Filter1/1
  Product3/1 -> Gain9/1
  Bus Selector6/2 -> abc to dq6/1  "<I>"
  [Io_d] -> Add2/2
  [Io_q] -> Add3/2
  [Vo_d] -> Filter/1
  Add4/1 -> Real-Imag to Complex1/1
  Real-Imag to Complex1/1 -> Complex to Magnitude-Angle1/1
  [Io_q] -> Gain7/1
  Complex to Magnitude-Angle1/1 -> Product3/1
  abc to dq6/1 -> Selector5/1
  In1/1 -> Add2/1  "Id_ref"
  Add9/1 -> Add8/2
  In2/1 -> Add3/1  "Iq_red"
  Constant4/1 -> Add9/3
  [Io_d] -> Gain8/1
  Gain/1 -> Add4/3
  Inport/1 -> Bus Selector6/1  "Bout"
  Gain10/1 -> Unit Delay1/1
  Demux5/1 -> [Io_d]
  Bus Creator/1 -> Outport/1  "m"
  [phi_d] -> Bus Creator/1  "phi_d"
  [phi_q] -> Bus Creator/2  "phi_q"
  [e_d] -> Bus Creator/3  "e_d"
  [e_q] -> Bus Creator/4  "e_q"
  [Io_d] -> Bus Creator/5  "i_d"
  [Io_q] -> Bus Creator/6  "i_q"
  Inport1/1 -> [wt]  "wt"
  Integrator/1 -> [phi_d], Gain1/1
  Gain1/1 -> Add4/4
  Integrator1/1 -> Gain3/1, [phi_q]
  Filter1/1 -> [e_q], Add5/4
  Gain8/1 -> Add5/3
  Gain2/1 -> Add5/1
  Add3/1 -> Integrator1/1, Gain2/1
  Gain3/1 -> Add5/2
  abc to dq1/1 -> Selector1/1
  Demux1/1 -> [Vo_d]
  Selector1/1 -> Demux1/1
  Demux1/2 -> [Vo_q]
  Bus Selector6/1 -> abc to dq1/1  "<V>"
  [wt] -> abc to dq1/2
  connections:
  A/RConn1 -- Three-Phase Series RLC Branch1/RConn1
  C/RConn1 -- Three-Phase Series RLC Branch1/RConn3
  DC Voltage Source2/LConn1 -- G/RConn1 -- DC Voltage Source1/RConn1
  Three-Phase Series RLC Branch1/LConn1 -- VSC (Average Model)/LConn1
  DC Voltage Source1/LConn1 -- VSC (Average Model)/RConn2
  B/RConn1 -- Three-Phase Series RLC Branch1/RConn2
  VSC (Average Model)/RConn1 -- DC Voltage Source2/RConn1
  Three-Phase Series RLC Branch1/LConn3 -- VSC (Average Model)/LConn3
  VSC (Average Model)/LConn2 -- Three-Phase Series RLC Branch1/LConn2

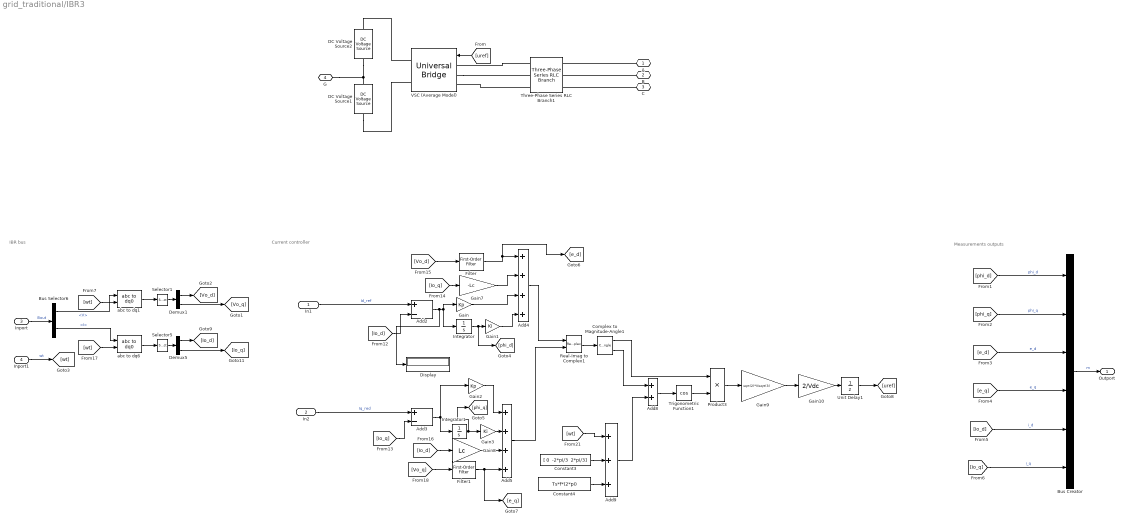
== system grid_traditional/IBR3 ==
  note: IBR bus
  note: Current controller
  note: Measurements outputs
  In1 : Inport
  In2 : Inport  Port=2
  Inport : Inport  Port=3
  Inport1 : Inport  Port=4
  Add2 : Sum  Inputs=+-
  Add3 : Sum  Inputs=+-
  Add4 : Sum  Inputs=++++
  Add5 : Sum  Inputs=++++
  Add8 : Sum
  Add9 : Sum  Inputs=+++
  Bus Creator : BusCreator  Inputs=6
  Bus Selector6 : BusSelector  OutputSignals=V,I
  Complex to Magnitude-Angle1 : ComplexToMagnitudeAngle
  Constant3 : Constant  Value="[ 0  -2*pi/3  2*pi/3]"
  Constant4 : Constant  Value=Ts*f*(2*pi)
  DC Voltage Source1 : spsDCVoltageSourceLib/DC Voltage Source  Amplitude=Vdc/2  Measurements=None
  DC Voltage Source2 : spsDCVoltageSourceLib/DC Voltage Source  Amplitude=Vdc/2  Measurements=None
  Demux1 : Demux  Outputs=2
  Demux5 : Demux  Outputs=2
  Display : Display
  Filter : spsFirstOrderFilterLib/First-Order Filter  FilterType=Lowpass  Tc=Tf  Ts=Ts  Initialize=on  Vac_Init=[0, 0, f]  Vdc_Init=0  PlotResponse=off  FreqRange="[0,  200,  1]"
  Filter1 : spsFirstOrderFilterLib/First-Order Filter  FilterType=Lowpass  Tc=Tf  Ts=Ts  Initialize=on  Vac_Init=[0, 0, f]  Vdc_Init=0  PlotResponse=off  FreqRange="[0,  200,  1]"
  Gain : Gain  Gain=Kp
  Gain1 : Gain  Gain=Ki
  Gain10 : Gain  Gain=2/Vdc
  Gain2 : Gain  Gain=Kp
  Gain3 : Gain  Gain=Ki
  Gain7 : Gain  Gain=-Lc
  Gain8 : Gain  Gain=Lc
  Gain9 : Gain  Gain=sqrt(2)*V/sqrt(3)
  Integrator : Integrator
  Integrator1 : Integrator
  Product3 : Product  Inputs=**  RndMeth=Zero
  Real-Imag to Complex1 : RealImagToComplex
  Selector1 : Selector  InputPortWidth=3  IndexOptions=Index vector (dialog)  Indices=[1 2]  OutputSizes=1
  Selector5 : Selector  InputPortWidth=3  IndexOptions=Index vector (dialog)  Indices=[1 2]  OutputSizes=1
  Three-Phase Series RLC Branch1 : spsThreePhaseSeriesRLCBranchLib/Three-Phase Series RLC Branch  LConnTagsString=A|B|C  RConnTagsString=A|B|C  BranchType=RL  Resistance=Rf*V^2/S  Inductance=Lf*V^2/S*1/(2*pi*f)  Capacitance=1e-6  Measurements=None
  Trigonometric Function1 : Trigonometry  Operator=cos
  Unit Delay1 : UnitDelay  SampleTime=Ts  HasFrameUpgradeWarning=on
  VSC (Average Model) : spsUniversalBridgeLib/Universal Bridge  Arms=3  SnubberResistance=1e5  SnubberCapacitance=inf  Device=Average-model based VSC  Ron=1e-3  Lon=0  ForwardVoltages="[  0  0  ]"  ForwardVoltage=0  GTOparameters=[ 10e-6 , 20e-6 ]  IGBTparameters=[ 1e-6 , 2e-6 ]  Measurements=None  Measurements_2=None  converterType=Rectifier
  abc to dq1 : spsabctodq0Lib/abc to dq0  Alignment=Aligned with phase A axis
  abc to dq6 : spsabctodq0Lib/abc to dq0  Alignment=Aligned with phase A axis
  A : PMIOPort  Side=Right
  B : PMIOPort  Port=2  Side=Right
  C : PMIOPort  Port=3  Side=Right
  G : PMIOPort  Port=4  Side=Left
  Outport : Outport
  wires:
  Add8/1 -> Trigonometric Function1/1
  [uref] -> VSC (Average Model)/1
  Add5/1 -> Real-Imag to Complex1/2
  Constant3/1 -> Add9/2
  Gain9/1 -> Gain10/1
  Gain7/1 -> Add4/2
  Unit Delay1/1 -> [uref]
  Trigonometric Function1/1 -> Product3/2
  [wt] -> Add9/1
  Complex to Magnitude-Angle1/2 -> Add8/1
  Add2/1 -> Display/1, Gain/1, Integrator/1
  Selector5/1 -> Demux5/1
  Demux5/2 -> [Io_q]
  [wt] -> abc to dq6/2
  Filter/1 -> [e_d], Add4/1
  [Vo_q] -> Filter1/1
  Product3/1 -> Gain9/1
  Bus Selector6/2 -> abc to dq6/1  "<I>"
  [Io_d] -> Add2/2
  [Io_q] -> Add3/2
  [Vo_d] -> Filter/1
  Add4/1 -> Real-Imag to Complex1/1
  Real-Imag to Complex1/1 -> Complex to Magnitude-Angle1/1
  [Io_q] -> Gain7/1
  Complex to Magnitude-Angle1/1 -> Product3/1
  abc to dq6/1 -> Selector5/1
  In1/1 -> Add2/1  "Id_ref"
  Add9/1 -> Add8/2
  In2/1 -> Add3/1  "Iq_red"
  Constant4/1 -> Add9/3
  [Io_d] -> Gain8/1
  Gain/1 -> Add4/3
  Inport/1 -> Bus Selector6/1  "Bout"
  Gain10/1 -> Unit Delay1/1
  Demux5/1 -> [Io_d]
  Bus Creator/1 -> Outport/1  "m"
  [phi_d] -> Bus Creator/1  "phi_d"
  [phi_q] -> Bus Creator/2  "phi_q"
  [e_d] -> Bus Creator/3  "e_d"
  [e_q] -> Bus Creator/4  "e_q"
  [Io_d] -> Bus Creator/5  "i_d"
  [Io_q] -> Bus Creator/6  "i_q"
  Inport1/1 -> [wt]  "wt"
  Integrator/1 -> [phi_d], Gain1/1
  Gain1/1 -> Add4/4
  Integrator1/1 -> Gain3/1, [phi_q]
  Filter1/1 -> [e_q], Add5/4
  Gain8/1 -> Add5/3
  Gain2/1 -> Add5/1
  Add3/1 -> Integrator1/1, Gain2/1
  Gain3/1 -> Add5/2
  abc to dq1/1 -> Selector1/1
  Demux1/1 -> [Vo_d]
  Selector1/1 -> Demux1/1
  Demux1/2 -> [Vo_q]
  Bus Selector6/1 -> abc to dq1/1  "<V>"
  [wt] -> abc to dq1/2
  connections:
  A/RConn1 -- Three-Phase Series RLC Branch1/RConn1
  C/RConn1 -- Three-Phase Series RLC Branch1/RConn3
  DC Voltage Source2/LConn1 -- G/RConn1 -- DC Voltage Source1/RConn1
  Three-Phase Series RLC Branch1/LConn1 -- VSC (Average Model)/LConn1
  DC Voltage Source1/LConn1 -- VSC (Average Model)/RConn2
  B/RConn1 -- Three-Phase Series RLC Branch1/RConn2
  VSC (Average Model)/RConn1 -- DC Voltage Source2/RConn1
  Three-Phase Series RLC Branch1/LConn3 -- VSC (Average Model)/LConn3
  VSC (Average Model)/LConn2 -- Three-Phase Series RLC Branch1/LConn2

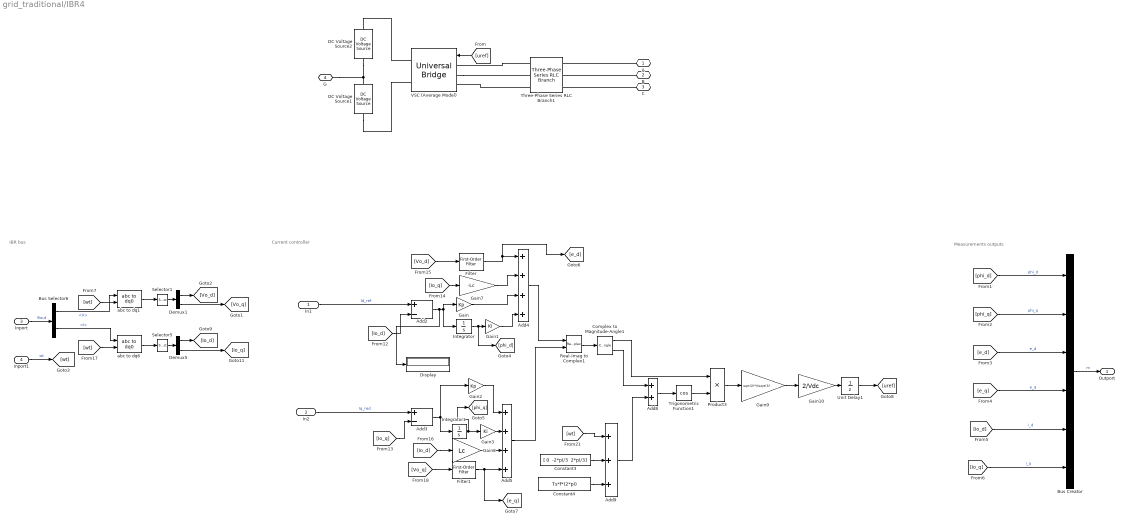
== system grid_traditional/IBR4 ==
  note: IBR bus
  note: Current controller
  note: Measurements outputs
  In1 : Inport
  In2 : Inport  Port=2
  Inport : Inport  Port=3
  Inport1 : Inport  Port=4
  Add2 : Sum  Inputs=+-
  Add3 : Sum  Inputs=+-
  Add4 : Sum  Inputs=++++
  Add5 : Sum  Inputs=++++
  Add8 : Sum
  Add9 : Sum  Inputs=+++
  Bus Creator : BusCreator  Inputs=6
  Bus Selector6 : BusSelector  OutputSignals=V,I
  Complex to Magnitude-Angle1 : ComplexToMagnitudeAngle
  Constant3 : Constant  Value="[ 0  -2*pi/3  2*pi/3]"
  Constant4 : Constant  Value=Ts*f*(2*pi)
  DC Voltage Source1 : spsDCVoltageSourceLib/DC Voltage Source  Amplitude=Vdc/2  Measurements=None
  DC Voltage Source2 : spsDCVoltageSourceLib/DC Voltage Source  Amplitude=Vdc/2  Measurements=None
  Demux1 : Demux  Outputs=2
  Demux5 : Demux  Outputs=2
  Display : Display
  Filter : spsFirstOrderFilterLib/First-Order Filter  FilterType=Lowpass  Tc=Tf  Ts=Ts  Initialize=on  Vac_Init=[0, 0, f]  Vdc_Init=0  PlotResponse=off  FreqRange="[0,  200,  1]"
  Filter1 : spsFirstOrderFilterLib/First-Order Filter  FilterType=Lowpass  Tc=Tf  Ts=Ts  Initialize=on  Vac_Init=[0, 0, f]  Vdc_Init=0  PlotResponse=off  FreqRange="[0,  200,  1]"
  Gain : Gain  Gain=Kp
  Gain1 : Gain  Gain=Ki
  Gain10 : Gain  Gain=2/Vdc
  Gain2 : Gain  Gain=Kp
  Gain3 : Gain  Gain=Ki
  Gain7 : Gain  Gain=-Lc
  Gain8 : Gain  Gain=Lc
  Gain9 : Gain  Gain=sqrt(2)*V/sqrt(3)
  Integrator : Integrator
  Integrator1 : Integrator
  Product3 : Product  Inputs=**  RndMeth=Zero
  Real-Imag to Complex1 : RealImagToComplex
  Selector1 : Selector  InputPortWidth=3  IndexOptions=Index vector (dialog)  Indices=[1 2]  OutputSizes=1
  Selector5 : Selector  InputPortWidth=3  IndexOptions=Index vector (dialog)  Indices=[1 2]  OutputSizes=1
  Three-Phase Series RLC Branch1 : spsThreePhaseSeriesRLCBranchLib/Three-Phase Series RLC Branch  LConnTagsString=A|B|C  RConnTagsString=A|B|C  BranchType=RL  Resistance=Rf*V^2/S  Inductance=Lf*V^2/S*1/(2*pi*f)  Capacitance=1e-6  Measurements=None
  Trigonometric Function1 : Trigonometry  Operator=cos
  Unit Delay1 : UnitDelay  SampleTime=Ts  HasFrameUpgradeWarning=on
  VSC (Average Model) : spsUniversalBridgeLib/Universal Bridge  Arms=3  SnubberResistance=1e5  SnubberCapacitance=inf  Device=Average-model based VSC  Ron=1e-3  Lon=0  ForwardVoltages="[  0  0  ]"  ForwardVoltage=0  GTOparameters=[ 10e-6 , 20e-6 ]  IGBTparameters=[ 1e-6 , 2e-6 ]  Measurements=None  Measurements_2=None  converterType=Rectifier
  abc to dq1 : spsabctodq0Lib/abc to dq0  Alignment=Aligned with phase A axis
  abc to dq6 : spsabctodq0Lib/abc to dq0  Alignment=Aligned with phase A axis
  A : PMIOPort  Side=Right
  B : PMIOPort  Port=2  Side=Right
  C : PMIOPort  Port=3  Side=Right
  G : PMIOPort  Port=4  Side=Left
  Outport : Outport
  wires:
  Add8/1 -> Trigonometric Function1/1
  [uref] -> VSC (Average Model)/1
  Add5/1 -> Real-Imag to Complex1/2
  Constant3/1 -> Add9/2
  Gain9/1 -> Gain10/1
  Gain7/1 -> Add4/2
  Unit Delay1/1 -> [uref]
  Trigonometric Function1/1 -> Product3/2
  [wt] -> Add9/1
  Complex to Magnitude-Angle1/2 -> Add8/1
  Add2/1 -> Display/1, Gain/1, Integrator/1
  Selector5/1 -> Demux5/1
  Demux5/2 -> [Io_q]
  [wt] -> abc to dq6/2
  Filter/1 -> [e_d], Add4/1
  [Vo_q] -> Filter1/1
  Product3/1 -> Gain9/1
  Bus Selector6/2 -> abc to dq6/1  "<I>"
  [Io_d] -> Add2/2
  [Io_q] -> Add3/2
  [Vo_d] -> Filter/1
  Add4/1 -> Real-Imag to Complex1/1
  Real-Imag to Complex1/1 -> Complex to Magnitude-Angle1/1
  [Io_q] -> Gain7/1
  Complex to Magnitude-Angle1/1 -> Product3/1
  abc to dq6/1 -> Selector5/1
  In1/1 -> Add2/1  "Id_ref"
  Add9/1 -> Add8/2
  In2/1 -> Add3/1  "Iq_red"
  Constant4/1 -> Add9/3
  [Io_d] -> Gain8/1
  Gain/1 -> Add4/3
  Inport/1 -> Bus Selector6/1  "Bout"
  Gain10/1 -> Unit Delay1/1
  Demux5/1 -> [Io_d]
  Bus Creator/1 -> Outport/1  "m"
  [phi_d] -> Bus Creator/1  "phi_d"
  [phi_q] -> Bus Creator/2  "phi_q"
  [e_d] -> Bus Creator/3  "e_d"
  [e_q] -> Bus Creator/4  "e_q"
  [Io_d] -> Bus Creator/5  "i_d"
  [Io_q] -> Bus Creator/6  "i_q"
  Inport1/1 -> [wt]  "wt"
  Integrator/1 -> [phi_d], Gain1/1
  Gain1/1 -> Add4/4
  Integrator1/1 -> Gain3/1, [phi_q]
  Filter1/1 -> [e_q], Add5/4
  Gain8/1 -> Add5/3
  Gain2/1 -> Add5/1
  Add3/1 -> Integrator1/1, Gain2/1
  Gain3/1 -> Add5/2
  abc to dq1/1 -> Selector1/1
  Demux1/1 -> [Vo_d]
  Selector1/1 -> Demux1/1
  Demux1/2 -> [Vo_q]
  Bus Selector6/1 -> abc to dq1/1  "<V>"
  [wt] -> abc to dq1/2
  connections:
  A/RConn1 -- Three-Phase Series RLC Branch1/RConn1
  C/RConn1 -- Three-Phase Series RLC Branch1/RConn3
  DC Voltage Source2/LConn1 -- G/RConn1 -- DC Voltage Source1/RConn1
  Three-Phase Series RLC Branch1/LConn1 -- VSC (Average Model)/LConn1
  DC Voltage Source1/LConn1 -- VSC (Average Model)/RConn2
  B/RConn1 -- Three-Phase Series RLC Branch1/RConn2
  VSC (Average Model)/RConn1 -- DC Voltage Source2/RConn1
  Three-Phase Series RLC Branch1/LConn3 -- VSC (Average Model)/LConn3
  VSC (Average Model)/LConn2 -- Three-Phase Series RLC Branch1/LConn2

== system grid_traditional/PLL (3ph) ==
  abc : Inport  PortDimensions=3  SampleTime=Ts
  Model : spsPLL3phModel/Discrete  SystemSampleTime=-1  VariantActivationTime=update diagram  AllowFlexibleInterface=on  Latency=0  AutoFrameSizeCalculation=off
      link override abc to dq0: Alignment=Aligned with phase A axis
  Freq : Outport  SampleTime=Ts  VectorParamsAs1DForOutWhenUnconnected=off
  wt : Outport  Port=2  SampleTime=Ts  VectorParamsAs1DForOutWhenUnconnected=off
  wires:
  Model/2 -> wt/1
  Model/1 -> Freq/1
  abc/1 -> Model/1

== system grid_traditional/PLL (3ph)1 ==
  abc : Inport  PortDimensions=3  SampleTime=Ts
  Model : spsPLL3phModel/Discrete  SystemSampleTime=-1  VariantActivationTime=update diagram  AllowFlexibleInterface=on  Latency=0  AutoFrameSizeCalculation=off
      link override abc to dq0: Alignment=Aligned with phase A axis
  Freq : Outport  SampleTime=Ts  VectorParamsAs1DForOutWhenUnconnected=off
  wt : Outport  Port=2  SampleTime=Ts  VectorParamsAs1DForOutWhenUnconnected=off
  wires:
  Model/2 -> wt/1
  Model/1 -> Freq/1
  abc/1 -> Model/1

== system grid_traditional/PLL (3ph)2 ==
  abc : Inport  PortDimensions=3  SampleTime=Ts
  Model : spsPLL3phModel/Discrete  SystemSampleTime=-1  VariantActivationTime=update diagram  AllowFlexibleInterface=on  Latency=0  AutoFrameSizeCalculation=off
      link override abc to dq0: Alignment=Aligned with phase A axis
  Freq : Outport  SampleTime=Ts  VectorParamsAs1DForOutWhenUnconnected=off
  wt : Outport  Port=2  SampleTime=Ts  VectorParamsAs1DForOutWhenUnconnected=off
  wires:
  Model/2 -> wt/1
  Model/1 -> Freq/1
  abc/1 -> Model/1

== system grid_traditional/PLL (3ph)3 ==
  abc : Inport  PortDimensions=3  SampleTime=Ts
  Model : spsPLL3phModel/Discrete  SystemSampleTime=-1  VariantActivationTime=update diagram  AllowFlexibleInterface=on  Latency=0  AutoFrameSizeCalculation=off
      link override abc to dq0: Alignment=Aligned with phase A axis
  Freq : Outport  SampleTime=Ts  VectorParamsAs1DForOutWhenUnconnected=off
  wt : Outport  Port=2  SampleTime=Ts  VectorParamsAs1DForOutWhenUnconnected=off
  wires:
  Model/2 -> wt/1
  Model/1 -> Freq/1
  abc/1 -> Model/1

== system grid_traditional/B1_IBR1/Subsystem ==
  V : Inport
  I : Inport  Port=2
  Enable : EnablePort
  Gain : Gain  Gain=2/3
  Gain1 : Gain  Gain=2/3
  power_calculation : spsPowerPositiveSequenceLib/Power (Positive-Sequence)  Freq=f  Vinit=[1, 0]  Iinit=[0, 0]  Ts=Ts
  P : Outport
  Q : Outport  Port=2
  wires:
  Gain1/1 -> Q/1  "Q"
  power_calculation/1 -> Gain/1
  Gain/1 -> P/1  "P"
  V/1 -> power_calculation/1
  I/1 -> power_calculation/2
  power_calculation/2 -> Gain1/1

== system grid_traditional/B1_SG1/Subsystem ==
  V : Inport
  I : Inport  Port=2
  Enable : EnablePort
  Gain : Gain  Gain=2/3
  Gain1 : Gain  Gain=2/3
  power_calculation : spsPowerPositiveSequenceLib/Power (Positive-Sequence)  Freq=f  Vinit=[1, 0]  Iinit=[0, 0]  Ts=Ts
  P : Outport
  Q : Outport  Port=2
  wires:
  Gain1/1 -> Q/1  "Q"
  power_calculation/1 -> Gain/1
  Gain/1 -> P/1  "P"
  V/1 -> power_calculation/1
  I/1 -> power_calculation/2
  power_calculation/2 -> Gain1/1

== system grid_traditional/B5_L/Subsystem ==
  V : Inport
  I : Inport  Port=2
  Enable : EnablePort
  Gain : Gain  Gain=2/3
  Gain1 : Gain  Gain=2/3
  power_calculation : spsPowerPositiveSequenceLib/Power (Positive-Sequence)  Freq=f  Vinit=[1, 0]  Iinit=[0, 0]  Ts=Ts
  P : Outport
  Q : Outport  Port=2
  wires:
  Gain1/1 -> Q/1  "Q"
  power_calculation/1 -> Gain/1
  Gain/1 -> P/1  "P"
  V/1 -> power_calculation/1
  I/1 -> power_calculation/2
  power_calculation/2 -> Gain1/1

== system grid_traditional/B5_SG6/Subsystem ==
  V : Inport
  I : Inport  Port=2
  Enable : EnablePort
  Gain : Gain  Gain=2/3
  Gain1 : Gain  Gain=2/3
  power_calculation : spsPowerPositiveSequenceLib/Power (Positive-Sequence)  Freq=f  Vinit=[1, 0]  Iinit=[0, 0]  Ts=Ts
  P : Outport
  Q : Outport  Port=2
  wires:
  Gain1/1 -> Q/1  "Q"
  power_calculation/1 -> Gain/1
  Gain/1 -> P/1  "P"
  V/1 -> power_calculation/1
  I/1 -> power_calculation/2
  power_calculation/2 -> Gain1/1

== system grid_traditional/B6_IBR3/Subsystem ==
  V : Inport
  I : Inport  Port=2
  Enable : EnablePort
  Gain : Gain  Gain=2/3
  Gain1 : Gain  Gain=2/3
  power_calculation : spsPowerPositiveSequenceLib/Power (Positive-Sequence)  Freq=f  Vinit=[1, 0]  Iinit=[0, 0]  Ts=Ts
  P : Outport
  Q : Outport  Port=2
  wires:
  Gain1/1 -> Q/1  "Q"
  power_calculation/1 -> Gain/1
  Gain/1 -> P/1  "P"
  V/1 -> power_calculation/1
  I/1 -> power_calculation/2
  power_calculation/2 -> Gain1/1

== system grid_traditional/B6_SG5/Subsystem ==
  V : Inport
  I : Inport  Port=2
  Enable : EnablePort
  Gain : Gain  Gain=2/3
  Gain1 : Gain  Gain=2/3
  power_calculation : spsPowerPositiveSequenceLib/Power (Positive-Sequence)  Freq=f  Vinit=[1, 0]  Iinit=[0, 0]  Ts=Ts
  P : Outport
  Q : Outport  Port=2
  wires:
  Gain1/1 -> Q/1  "Q"
  power_calculation/1 -> Gain/1
  Gain/1 -> P/1  "P"
  V/1 -> power_calculation/1
  I/1 -> power_calculation/2
  power_calculation/2 -> Gain1/1

== system grid_traditional/B7_IBR4/Subsystem ==
  V : Inport
  I : Inport  Port=2
  Enable : EnablePort
  Gain : Gain  Gain=2/3
  Gain1 : Gain  Gain=2/3
  power_calculation : spsPowerPositiveSequenceLib/Power (Positive-Sequence)  Freq=f  Vinit=[1, 0]  Iinit=[0, 0]  Ts=Ts
  P : Outport
  Q : Outport  Port=2
  wires:
  Gain1/1 -> Q/1  "Q"
  power_calculation/1 -> Gain/1
  Gain/1 -> P/1  "P"
  V/1 -> power_calculation/1
  I/1 -> power_calculation/2
  power_calculation/2 -> Gain1/1

== system grid_traditional/B7_L/Subsystem ==
  V : Inport
  I : Inport  Port=2
  Enable : EnablePort
  Gain : Gain  Gain=2/3
  Gain1 : Gain  Gain=2/3
  power_calculation : spsPowerPositiveSequenceLib/Power (Positive-Sequence)  Freq=f  Vinit=[1, 0]  Iinit=[0, 0]  Ts=Ts
  P : Outport
  Q : Outport  Port=2
  wires:
  Gain1/1 -> Q/1  "Q"
  power_calculation/1 -> Gain/1
  Gain/1 -> P/1  "P"
  V/1 -> power_calculation/1
  I/1 -> power_calculation/2
  power_calculation/2 -> Gain1/1

== system grid_traditional/B7_SG4/Subsystem ==
  V : Inport
  I : Inport  Port=2
  Enable : EnablePort
  Gain : Gain  Gain=2/3
  Gain1 : Gain  Gain=2/3
  power_calculation : spsPowerPositiveSequenceLib/Power (Positive-Sequence)  Freq=f  Vinit=[1, 0]  Iinit=[0, 0]  Ts=Ts
  P : Outport
  Q : Outport  Port=2
  wires:
  Gain1/1 -> Q/1  "Q"
  power_calculation/1 -> Gain/1
  Gain/1 -> P/1  "P"
  V/1 -> power_calculation/1
  I/1 -> power_calculation/2
  power_calculation/2 -> Gain1/1

== system grid_traditional/B8_IBR2/Subsystem ==
  V : Inport
  I : Inport  Port=2
  Enable : EnablePort
  Gain : Gain  Gain=2/3
  Gain1 : Gain  Gain=2/3
  power_calculation : spsPowerPositiveSequenceLib/Power (Positive-Sequence)  Freq=f  Vinit=[1, 0]  Iinit=[0, 0]  Ts=Ts
  P : Outport
  Q : Outport  Port=2
  wires:
  Gain1/1 -> Q/1  "Q"
  power_calculation/1 -> Gain/1
  Gain/1 -> P/1  "P"
  V/1 -> power_calculation/1
  I/1 -> power_calculation/2
  power_calculation/2 -> Gain1/1

== system grid_traditional/B8_SG3/Subsystem ==
  V : Inport
  I : Inport  Port=2
  Enable : EnablePort
  Gain : Gain  Gain=2/3
  Gain1 : Gain  Gain=2/3
  power_calculation : spsPowerPositiveSequenceLib/Power (Positive-Sequence)  Freq=f  Vinit=[1, 0]  Iinit=[0, 0]  Ts=Ts
  P : Outport
  Q : Outport  Port=2
  wires:
  Gain1/1 -> Q/1  "Q"
  power_calculation/1 -> Gain/1
  Gain/1 -> P/1  "P"
  V/1 -> power_calculation/1
  I/1 -> power_calculation/2
  power_calculation/2 -> Gain1/1

== system grid_traditional/B9_L/Subsystem ==
  V : Inport
  I : Inport  Port=2
  Enable : EnablePort
  Gain : Gain  Gain=2/3
  Gain1 : Gain  Gain=2/3
  power_calculation : spsPowerPositiveSequenceLib/Power (Positive-Sequence)  Freq=f  Vinit=[1, 0]  Iinit=[0, 0]  Ts=Ts
  P : Outport
  Q : Outport  Port=2
  wires:
  Gain1/1 -> Q/1  "Q"
  power_calculation/1 -> Gain/1
  Gain/1 -> P/1  "P"
  V/1 -> power_calculation/1
  I/1 -> power_calculation/2
  power_calculation/2 -> Gain1/1

== system grid_traditional/B9_SG2/Subsystem ==
  V : Inport
  I : Inport  Port=2
  Enable : EnablePort
  Gain : Gain  Gain=2/3
  Gain1 : Gain  Gain=2/3
  power_calculation : spsPowerPositiveSequenceLib/Power (Positive-Sequence)  Freq=f  Vinit=[1, 0]  Iinit=[0, 0]  Ts=Ts
  P : Outport
  Q : Outport  Port=2
  wires:
  Gain1/1 -> Q/1  "Q"
  power_calculation/1 -> Gain/1
  Gain/1 -> P/1  "P"
  V/1 -> power_calculation/1
  I/1 -> power_calculation/2
  power_calculation/2 -> Gain1/1
